simulink model "sensor_redundancy_manager_wrapper"  (R2023b)
settings: Solver=FixedStepAuto  StartTime=0.0  StopTime=10.0  RelTol=1e-3
settings Model: Creator=Aniket  LastModifiedBy=Aniket
settings ConfigComp: DVTestSuiteOptimization=Auto  DVDetectOutOfBounds=on  DVModelReferenceHarness=on  DVHarnessSource=Signal Editor  DVRebuildModelRepresentation=IfChangeIsDetected

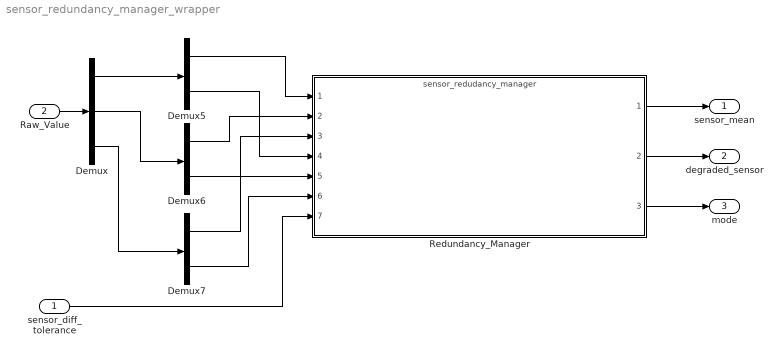
== system sensor_redundancy_manager_wrapper ==
  sensor_diff_tolerance : Inport
  Raw_Value : Inport  Port=2
  Demux : Demux  Outputs=3
  Demux5 : Demux  Outputs=2
  Demux6 : Demux  Outputs=2
  Demux7 : Demux  Outputs=2
  Redundancy_Manager : ModelReference  ModelNameDialog=sensor_redudancy_manager.mdl  SimulationMode=Normal  ModelReferenceVersion=1.19
  sensor_mean : Outport
  degraded_sensor : Outport  Port=2
  mode : Outport  Port=3
  wires:
  Demux/2 -> Demux6/1
  Redundancy_Manager/1 -> sensor_mean/1
  Redundancy_Manager/3 -> mode/1
  Redundancy_Manager/2 -> degraded_sensor/1
  sensor_diff_tolerance/1 -> Redundancy_Manager/7
  Demux7/2 -> Redundancy_Manager/6
  Demux7/1 -> Redundancy_Manager/3
  Demux5/1 -> Redundancy_Manager/1
  Demux6/1 -> Redundancy_Manager/2
  Raw_Value/1 -> Demux/1
  Demux/3 -> Demux7/1
  Demux6/2 -> Redundancy_Manager/5
  Demux/1 -> Demux5/1
  Demux5/2 -> Redundancy_Manager/4
